simulink model "lindiscrmodel_lqr_dd"  (R2019a)
settings: Solver=VariableStepAuto  StartTime=0.0  StopTime=30  RelTol=1e-3
InitFcn:
  | lindiscrmodel
values from neighbouring files (symbols this model uses):
  Ts = 0.01    [lindiscrmodel.m]
undefined symbols (not defined in the file or in its folder): Discrete, K1, linmat, Time
libraries: ctrlSharedLib x1
settings Model: Creator=jessi  LastModifiedBy=jessi

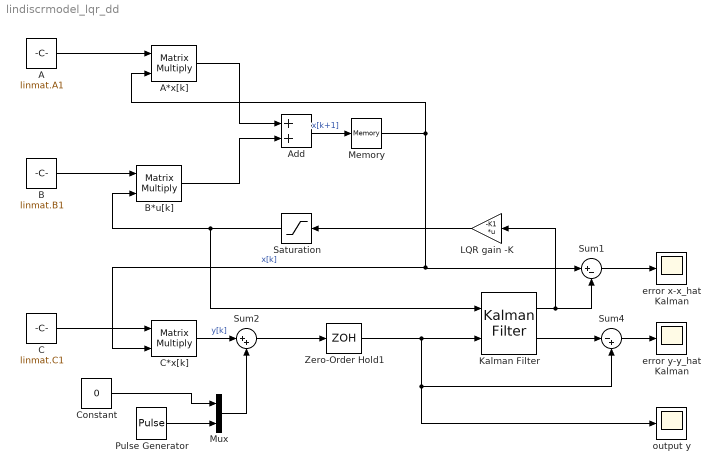
== system lindiscrmodel_lqr_dd ==
  A : Constant  Value=linmat.A1  SampleTime=Ts
  A*x[k] : Product  Multiplication=Matrix(*)
  Add : Sum
  B : Constant  Value=linmat.B1  SampleTime=Ts
  B*u[k] : Product  Multiplication=Matrix(*)
  C : Constant  Value=linmat.C1  SampleTime=Ts
  C*x[k] : Product  Multiplication=Matrix(*)
  Constant : Constant  Value=0  SampleTime=Ts
  Kalman Filter : ctrlSharedLib/Kalman Filter  TimeDomain=Discrete-Time  UseCurrentEstimator=on  ModelSource=Individual A, B, C, D matrices  ModelSourceVariable=sysd2  A=linmat.A1  B=linmat.B1  C=linmat.C1  D=linmat.D1  NumberOfStates=1  NumberOfInputs=1  NumberOfOutputs=1  InitialEstimateSource=Dialog  X0=[0.25*pi;0;0;0]  P0=10  UseK=off  UseGH=off  NumberOfProcessNoiseInputs=1  G=1  TimeInvariantG=on  H=0  TimeInvariantH=on  Q=diag([100 100 0.01 0.01])  TimeInvariantQ=on  R=0.0001  TimeInvariantR=on  N=0  TimeInvariantN=on  AddInputPort=on  AddEnablePort=off  OutputEstimatedY=on  OutputP=off  Ts=Ts
      settings: SourceProductBaseCode=CT
  LQR gain -K : Gain  Gain=-K1  Multiplication=Matrix(K*u)
  Memory : Memory  InitialCondition=[0.25*pi;0;0;0]
  Mux : Mux  Inputs=2
  Pulse Generator : DiscretePulseGenerator  PulseType=Time based  Amplitude=0  Period=10  PulseWidth=5
  Saturation : Saturate  UpperLimit=1  LowerLimit=-1
  Sum1 : Sum  Inputs=|+-
  Sum2 : Sum  Inputs=|++
  Sum4 : Sum  Inputs=|-+
  Zero-Order Hold1 : ZeroOrderHold  SampleTime=Ts
  error x-x_hat Kalman : Scope
  error y-y_hat Kalman : Scope
  output y : Scope
  wires:
  B/1 -> B*u[k]/1
  A/1 -> A*x[k]/1
  A*x[k]/1 -> Add/1
  B*u[k]/1 -> Add/2
  Memory/1 -> A*x[k]/2, Sum1/1, C*x[k]/2  "x[k]"
  C/1 -> C*x[k]/1
  Add/1 -> Memory/1  "x[k+1]"
  Sum1/1 -> error x-x_hat Kalman/1
  Kalman Filter/1 -> LQR gain -K/1, Sum1/2
  C*x[k]/1 -> Sum2/1  "y[k]"
  Sum4/1 -> error y-y_hat Kalman/1
  Sum2/1 -> Zero-Order Hold1/1
  Zero-Order Hold1/1 -> output y/1, Sum4/2, Kalman Filter/2
  LQR gain -K/1 -> Saturation/1
  Saturation/1 -> Kalman Filter/1, B*u[k]/2
  Kalman Filter/2 -> Sum4/1
  Pulse Generator/1 -> Mux/2
  Mux/1 -> Sum2/2
  Constant/1 -> Mux/1
